simulink model "open_loop_satellite_load"  (R2021a)
settings: Solver=ode45  StartTime=0.0  StopTime=100  RelTol=1e-3  EnableMultiTasking=on
values from neighbouring files (symbols this model uses):
  b = 10    [Lab_2.m]    (also in tutorialsatellite_student.m)
  Jt = J+Jm*N^2    (= 190)    [Lab_2.m]    (also in tutorialsatellite_student.m = 120)
  K = 10000    [Lab_2.m]
  ke = 0.2    [Lab_2.m]    (also in tutorialsatellite_student.m)
  km = 0.2    [Lab_2.m]    (also in tutorialsatellite_student.m)
  L = 0.002    [Lab_2.m]
  N = 300    [Lab_2.m]    (also in tutorialsatellite_student.m = 100)
  R = 2    [Lab_2.m]
settings Model: Creator=c.berard  LastModifiedBy=fades
settings SolverCC: AlgebraicLoopSolver=TrustRegion
settings DataIOCC: LimitDataPoints=on  SaveFormat=Array  SignalLoggingSaveFormat=ModelDataLogs  ReturnWorkspaceOutputs=off  SignalLoggingName=sigsOut
settings OptimizationCC: BlockReduction=off  BooleanDataType=off  ExpressionDepthLimit=2147483647  InitFltsAndDblsToZero=on  LifeSpan=inf
settings DebuggingCC: SaveWithParameterizedLinksMsg=none  UnderspecifiedInitializationDetection=Classic  MergeDetectMultiDrivingBlocksExec=none  SignalResolutionControl=TryResolveAllWithWarning  MultiTaskDSMMsg=warning  MultiTaskCondExecSysMsg=none  FcnCallInpInsideContextMsg=warning  AllowSymbolicDim=off  StateNameClashWarn=warning  SFUnexpectedBacktrackingDiag=warning  SFNoUnconditionalDefaultTransitionDiag=warning  SFExecutionAtInitializationDiag=none  SFMachineParentedDataDiag=warning  ArithmeticOperatorsInVariantConditions=warning
settings HardwareCC: ProdBitPerPointer=32  ProdBitPerSizeT=32  ProdBitPerPtrDiffT=32  ProdLargestAtomicFloat=None  ProdIntDivRoundTo=Undefined  ProdEndianess=Unspecified  ProdWordSize=32  ProdHWDeviceType=32-bit Generic  TargetUnknown=on
settings ModelReferenceCC: PropagateSignalLabelsOutOfModel=off
settings SFSimCC: SimUseLocalCustomCode=off  CustomCodeUndefinedFunction=UseInterfaceOnly
settings RTWCC: RTWUseLocalCustomCode=off
settings CodeAppCC: StateflowObjectComments=on
settings GRTTargetCC: TargetFcnLib=ansi_tfl_tmw.mat  TargetLangStandard=C89/C90 (ANSI)  CombineOutputUpdateFcns=off  GRTInterface=on
settings ConfigComp: CovMetricSettings=dw  CovSaveCumulativeToWorkspaceVar=on  CovSaveSingleToWorkspaceVar=on  CovExternalEMLEnable=off

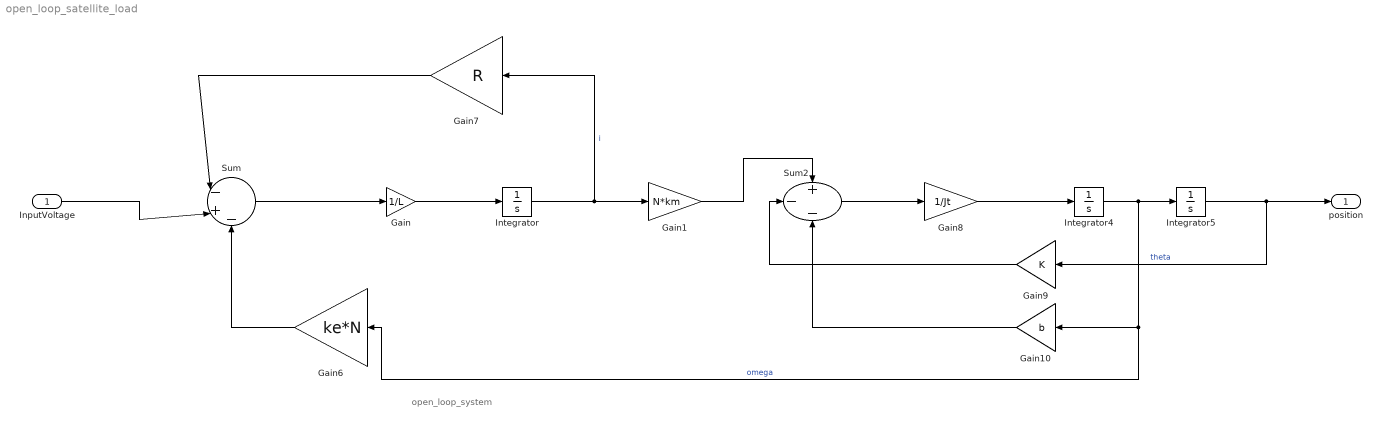
== system open_loop_satellite_load ==
  note: open_loop_system
  InputVoltage : Inport
  Gain : Gain  Gain=1/L
  Gain1 : Gain  Gain=N*km
  Gain10 : Gain  Gain=b
  Gain6 : Gain  Gain=ke*N
  Gain7 : Gain  Gain=R
  Gain8 : Gain  Gain=1/Jt
  Gain9 : Gain  Gain=K
  Integrator : Integrator
  Integrator4 : Integrator
  Integrator5 : Integrator
  Sum : Sum  Inputs=|-+-
  Sum2 : Sum  Inputs=+--
  position : Outport  VectorParamsAs1DForOutWhenUnconnected=off
  wires:
  InputVoltage/1 -> Sum/2
  Gain/1 -> Integrator/1
  Gain6/1 -> Sum/3
  Gain7/1 -> Sum/1
  Sum/1 -> Gain/1
  Integrator/1 -> Gain7/1, Gain1/1  "i"
  Gain1/1 -> Sum2/1
  Sum2/1 -> Gain8/1
  Gain8/1 -> Integrator4/1
  Integrator4/1 -> Gain10/1, Gain6/1, Integrator5/1  "omega"
  Gain9/1 -> Sum2/2
  Gain10/1 -> Sum2/3
  Integrator5/1 -> Gain9/1, position/1  "theta"
